simulink model "uavL1G"  (R2018b)
settings: Solver=VariableStepAuto  StartTime=0.0  StopTime=100  RelTol=1e-3
settings Model: Creator=win7-s  LastModifiedBy=JIA X S

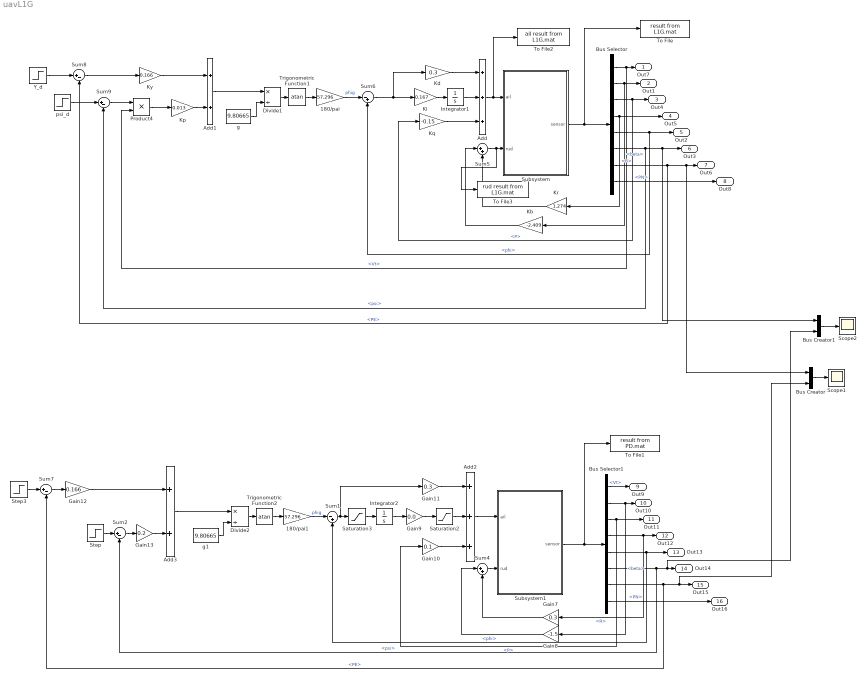
== system uavL1G ==
  180/pai : Gain  Gain=57.296
  180/pai1 : Gain  Gain=57.296
  Add : Sum  Inputs=+++
  Add1 : Sum
  Add2 : Sum  Inputs=+++
  Add3 : Sum
  Bus Creator : BusCreator  Inputs=2
  Bus Creator1 : BusCreator  Inputs=2
  Bus Selector : BusSelector  OutputSignals=Vt,beta,P,R,phi,psi,PE,PN
  Bus Selector1 : BusSelector  OutputSignals=Vt,beta,P,R,phi,psi,PE,PN
  Divide1 : Product  Inputs=*/
  Divide2 : Product  Inputs=*/
  Gain10 : Gain  Gain=0.1
  Gain11 : Gain  Gain=0.3
  Gain12 : Gain  Gain=0.166
  Gain13 : Gain  Gain=0.2
  Gain7 : Gain  Gain=0.3
  Gain8 : Gain  Gain=-1.5
  Gain9 : Gain  Gain=0.0
  Integrator1 : Integrator
  Integrator2 : Integrator
  Kb : Gain  Gain=-2.409
  Kd : Gain  Gain=0.3
  Ki : Gain  Gain=0.167
  Kp : Gain  Gain=0.013
  Kq : Gain  Gain=-0.15
  Kr : Gain  Gain=1.274
  Ky : Gain  Gain=0.166
  Product4 : Product
  Saturation2 : Saturate
  Saturation3 : Saturate
  Scope1 : Scope
  Scope2 : Scope
  Step : Step  Time=0  After=0  SampleTime=0
  Step3 : Step  Time=0  Before=5  After=5  SampleTime=0
  Subsystem : Subsystem
  Subsystem1 : Subsystem
  Sum1 : Sum  Inputs=|-+
  Sum{2,7..9} (4 alike) : Sum  Inputs=|+-
  Sum4 : Sum  Inputs=|++
  Sum5 : Sum  Inputs=|++
  Sum6 : Sum  Inputs=|-+
  To File : ToFile  Filename=result from L1G.mat  SaveFormat=Timeseries
  To File1 : ToFile  Filename=result from PD.mat  SaveFormat=Timeseries
  To File2 : ToFile  Filename=ail result from L1G.mat  SaveFormat=Timeseries
  To File3 : ToFile  Filename=rud result from L1G.mat  SaveFormat=Timeseries
  Trigonometric Function1 : Trigonometry  Operator=atan
  Trigonometric Function2 : Trigonometry  Operator=atan
  Y_d : Step  Time=0  Before=5  After=5  SampleTime=0
  g : Constant  Value=9.80665
  g1 : Constant  Value=9.80665
  psi_d : Step  Time=0  After=0  SampleTime=0
  Out7 : Outport
  Out1 : Outport  Port=2
  Out4 : Outport  Port=3
  Out5 : Outport  Port=4
  Out2 : Outport  Port=5
  Out3 : Outport  Port=6
  Out6 : Outport  Port=7
  Out8 : Outport  Port=8
  Out9 : Outport  Port=9
  Out10 : Outport  Port=10
  Out11 : Outport  Port=11
  Out12 : Outport  Port=12
  Out13 : Outport  Port=13
  Out14 : Outport  Port=14
  Out15 : Outport  Port=15
  Out16 : Outport  Port=16
  wires:
  Bus Selector/7 -> Bus Creator/1, Out6/1, Sum8/2  "<PE>"
  Bus Selector/3 -> Kq/1, Out4/1  "<P>"
  Bus Selector/6 -> Bus Creator1/1, Out3/1, Sum9/2  "<psi>"
  Bus Selector/2 -> Kb/1, Out1/1  "<beta>"
  Bus Selector/5 -> Sum6/2, Out2/1  "<phi>"
  Bus Selector/4 -> Out5/1, Kr/1  "<R>"
  Subsystem/1(sensor) -> To File/1, Bus Selector/1
  g/1 -> Divide1/2
  Divide1/1 -> Trigonometric Function1/1
  Ki/1 -> Integrator1/1
  Bus Selector/1 -> Product4/2, Out7/1  "<Vt>"
  Bus Selector/8 -> Out8/1  "<PN>"
  Integrator1/1 -> Add/2
  Kd/1 -> Add/1
  Kq/1 -> Add/3
  Kb/1 -> Sum5/1
  Kr/1 -> Sum5/2
  Sum6/1 -> Kd/1, Ki/1
  Trigonometric Function1/1 -> 180/pai/1
  Add/1 -> To File2/1, Subsystem/1(ail)
  Sum5/1 -> To File3/1, Subsystem/2(rud)
  Y_d/1 -> Sum8/1
  Ky/1 -> Add1/1
  Product4/1 -> Kp/1
  Sum8/1 -> Ky/1
  Sum9/1 -> Product4/1
  180/pai/1 -> Sum6/1  "phig"
  Kp/1 -> Add1/2
  Add1/1 -> Divide1/1
  psi_d/1 -> Sum9/1
  Bus Selector1/1 -> Out9/1  "<Vt>"
  Bus Selector1/8 -> Out16/1  "<PN>"
  Subsystem1/1(sensor) -> To File1/1, Bus Selector1/1
  Gain13/1 -> Add3/2
  Gain11/1 -> Add2/1
  Gain7/1 -> Sum4/2
  Bus Selector1/3 -> Out11/1, Gain10/1  "<P>"
  Bus Selector1/4 -> Gain7/1, Out12/1  "<R>"
  Gain9/1 -> Saturation2/1
  Sum2/1 -> Gain13/1
  Bus Selector1/6 -> Sum2/2, Bus Creator1/2, Out14/1  "<psi>"
  Bus Selector1/2 -> Gain8/1, Out10/1  "<beta>"
  Gain8/1 -> Sum4/1
  Bus Selector1/5 -> Sum1/2, Out13/1  "<phi>"
  Integrator2/1 -> Gain9/1
  Sum7/1 -> Gain12/1
  Saturation2/1 -> Add2/2
  Saturation3/1 -> Integrator2/1
  Step/1 -> Sum2/1
  Sum4/1 -> Subsystem1/2(rud)
  Gain10/1 -> Add2/3
  Bus Selector1/7 -> Sum7/2, Bus Creator/2, Out15/1  "<PE>"
  Step3/1 -> Sum7/1
  Gain12/1 -> Add3/1
  Sum1/1 -> Gain11/1, Saturation3/1
  Add2/1 -> Subsystem1/1(ail)
  Bus Creator/1 -> Scope1/1
  Bus Creator1/1 -> Scope2/1
  Add3/1 -> Divide2/1
  Trigonometric Function2/1 -> 180/pai1/1
  Divide2/1 -> Trigonometric Function2/1
  g1/1 -> Divide2/2
  180/pai1/1 -> Sum1/1  "phig"

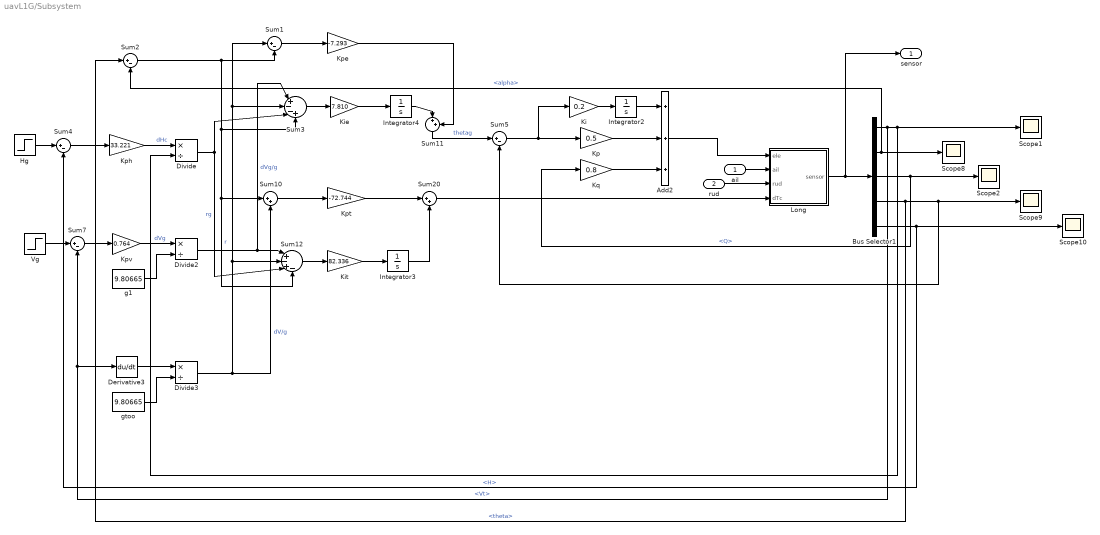
== system uavL1G/Subsystem ==
  ail : Inport
  rud : Inport  Port=2
  Add2 : Sum  Inputs=+++
  Bus Selector1 : BusSelector  OutputSignals=Vt,alpha,Q,theta,H
  Derivative3 : Derivative
  Divide : Product  Inputs=*/
  Divide2 : Product  Inputs=*/
  Divide3 : Product  Inputs=*/
  Hg : Step  Time=0  Before=100  After=100  SampleTime=0
  Integrator2 : Integrator
  Integrator3 : Integrator
  Integrator4 : Integrator
  Ki : Gain  Gain=0.2
  Kie : Gain  Gain=7.810
  Kit : Gain  Gain=82.336
  Kp : Gain  Gain=0.5
  Kpe : Gain  Gain=-7.293
  Kph : Gain  Gain=33.221
  Kpt : Gain  Gain=-72.744
  Kpv : Gain  Gain=0.764
  Kq : Gain  Gain=0.8
  Long : Subsystem
  Scope{1..2,8..10} (5 alike) : Scope
  Sum{1..2,4..5,7} (5 alike) : Sum  Inputs=|+-
  Sum10 : Sum  Inputs=|++
  Sum11 : Sum  Inputs=|++
  Sum12 : Sum  Inputs=|+-+-
  Sum20 : Sum  Inputs=|++
  Sum3 : Sum  Inputs=|+--+
  Vg : Step  Time=0  Before=20  After=20  SampleTime=0
  g1 : Constant  Value=9.80665
  gtoo : Constant  Value=9.80665
  sensor : Outport  VectorParamsAs1DForOutWhenUnconnected=on
  wires:
  Bus Selector1/3 -> Kq/1, Scope2/1  "<Q>"
  Sum10/1 -> Kpt/1
  Kq/1 -> Add2/3
  Divide3/1 -> Sum10/2, Sum12/2, Sum3/2, Sum1/1  "dV/g"
  Sum7/1 -> Kpv/1
  Sum4/1 -> Kph/1
  Integrator3/1 -> Sum20/2
  Bus Selector1/5 -> Sum4/2, Scope10/1  "<H>"
  Hg/1 -> Sum4/1
  Bus Selector1/1 -> Divide/2, Scope1/1, Sum7/2, Derivative3/1  "<Vt>"
  Kph/1 -> Divide/1  "dHc"
  gtoo/1 -> Divide3/2
  Sum1/1 -> Kpe/1
  Divide/1 -> Sum12/3, Sum3/3  "rg"
  Vg/1 -> Sum7/1
  Kpv/1 -> Divide2/1  "dVg"
  Integrator2/1 -> Add2/1
  Bus Selector1/4 -> Sum2/1, Sum5/2, Scope9/1  "<theta>"
  Divide2/1 -> Sum12/1, Sum3/1  "dVg/g"
  Ki/1 -> Integrator2/1
  Sum12/1 -> Kit/1
  Integrator4/1 -> Sum11/1
  Sum3/1 -> Kie/1
  Sum20/1 -> Long/4(dTc)
  Sum11/1 -> Sum5/1  "thetag"
  Derivative3/1 -> Divide3/1
  Kp/1 -> Add2/2
  Kit/1 -> Integrator3/1
  Long/1(sensor) -> sensor/1, Bus Selector1/1
  rud/1 -> Long/3(rud)
  Sum2/1 -> Sum12/4, Sum10/1, Sum3/4, Sum1/2  "r"
  ail/1 -> Long/2(ail)
  Kie/1 -> Integrator4/1
  Sum5/1 -> Ki/1, Kp/1
  Add2/1 -> Long/1(ele)
  Kpt/1 -> Sum20/1
  Bus Selector1/2 -> Scope8/1, Sum2/2  "<alpha>"
  Kpe/1 -> Sum11/2
  g1/1 -> Divide2/2

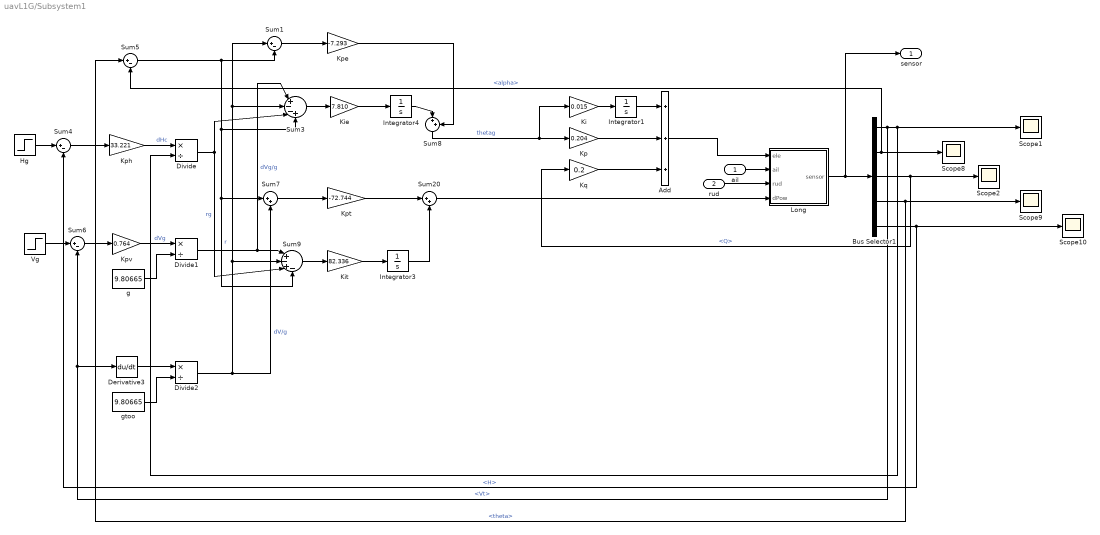
== system uavL1G/Subsystem1 ==
  ail : Inport
  rud : Inport  Port=2
  Add : Sum  Inputs=+++
  Bus Selector1 : BusSelector  OutputSignals=Vt,alpha,Q,theta,H
  Derivative3 : Derivative
  Divide : Product  Inputs=*/
  Divide1 : Product  Inputs=*/
  Divide2 : Product  Inputs=*/
  Hg : Step  Time=0  Before=100  After=100  SampleTime=0
  Integrator1 : Integrator
  Integrator3 : Integrator
  Integrator4 : Integrator
  Ki : Gain  Gain=0.015
  Kie : Gain  Gain=7.810
  Kit : Gain  Gain=82.336
  Kp : Gain  Gain=0.204
  Kpe : Gain  Gain=-7.293
  Kph : Gain  Gain=33.221
  Kpt : Gain  Gain=-72.744
  Kpv : Gain  Gain=0.764
  Kq : Gain  Gain=0.2
  Long : Subsystem
  Scope{1..2,8..10} (5 alike) : Scope
  Sum{1,4..6} (4 alike) : Sum  Inputs=|+-
  Sum20 : Sum  Inputs=|++
  Sum3 : Sum  Inputs=|+--+
  Sum7 : Sum  Inputs=|++
  Sum8 : Sum  Inputs=|++
  Sum9 : Sum  Inputs=|+-+-
  Vg : Step  Time=0  Before=20  After=20  SampleTime=0
  g : Constant  Value=9.80665
  gtoo : Constant  Value=9.80665
  sensor : Outport  VectorParamsAs1DForOutWhenUnconnected=on
  wires:
  Sum6/1 -> Kpv/1
  gtoo/1 -> Divide2/2
  Kie/1 -> Integrator4/1
  Integrator3/1 -> Sum20/2
  Sum8/1 -> Ki/1, Kp/1  "thetag"
  Ki/1 -> Integrator1/1
  Sum1/1 -> Kpe/1
  Sum9/1 -> Kit/1
  Kit/1 -> Integrator3/1
  Vg/1 -> Sum6/1
  Divide2/1 -> Sum7/2, Sum9/2, Sum3/2, Sum1/1  "dV/g"
  Kpv/1 -> Divide1/1  "dVg"
  Kpe/1 -> Sum8/2
  Hg/1 -> Sum4/1
  Divide/1 -> Sum9/3, Sum3/3  "rg"
  Long/1(sensor) -> sensor/1, Bus Selector1/1
  ail/1 -> Long/2(ail)
  Integrator4/1 -> Sum8/1
  Sum5/1 -> Sum9/4, Sum7/1, Sum3/4, Sum1/2  "r"
  Derivative3/1 -> Divide2/1
  rud/1 -> Long/3(rud)
  Divide1/1 -> Sum9/1, Sum3/1  "dVg/g"
  Bus Selector1/4 -> Sum5/1, Scope9/1  "<theta>"
  Sum3/1 -> Kie/1
  g/1 -> Divide1/2
  Sum7/1 -> Kpt/1
  Bus Selector1/1 -> Divide/2, Scope1/1, Sum6/2, Derivative3/1  "<Vt>"
  Kpt/1 -> Sum20/1
  Kph/1 -> Divide/1  "dHc"
  Bus Selector1/5 -> Sum4/2, Scope10/1  "<H>"
  Sum4/1 -> Kph/1
  Bus Selector1/3 -> Kq/1, Scope2/1  "<Q>"
  Sum20/1 -> Long/4(dPow)
  Bus Selector1/2 -> Scope8/1, Sum5/2  "<alpha>"
  Kp/1 -> Add/2
  Add/1 -> Long/1(ele)
  Kq/1 -> Add/3
  Integrator1/1 -> Add/1

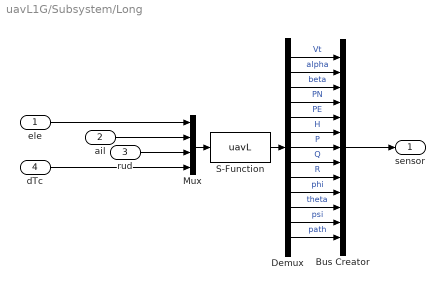
== system uavL1G/Subsystem/Long ==
  ele : Inport
  ail : Inport  Port=2
  rud : Inport  Port=3
  dTc : Inport  Port=4
  Bus Creator : BusCreator  Inputs=13
  Demux : Demux  Outputs=13
  Mux : Mux
  S-Function : S-Function  FunctionName=uavL  SFunctionDeploymentMode=off  EnableBusSupport=off
  sensor : Outport  VectorParamsAs1DForOutWhenUnconnected=on
  wires:
  Bus Creator/1 -> sensor/1
  ele/1 -> Mux/1
  rud/1 -> Mux/3
  Demux/12 -> Bus Creator/12  "psi"
  Mux/1 -> S-Function/1
  ail/1 -> Mux/2
  Demux/10 -> Bus Creator/10  "phi"
  Demux/13 -> Bus Creator/13  "path"
  Demux/5 -> Bus Creator/5  "PE"
  Demux/9 -> Bus Creator/9  "R"
  Demux/8 -> Bus Creator/8  "Q"
  Demux/7 -> Bus Creator/7  "P"
  Demux/6 -> Bus Creator/6  "H"
  Demux/2 -> Bus Creator/2  "alpha"
  Demux/3 -> Bus Creator/3  "beta"
  Demux/11 -> Bus Creator/11  "theta"
  Demux/4 -> Bus Creator/4  "PN"
  Demux/1 -> Bus Creator/1  "Vt"
  dTc/1 -> Mux/4
  S-Function/1 -> Demux/1

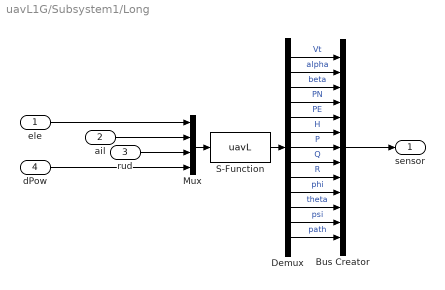
== system uavL1G/Subsystem1/Long ==
  ele : Inport
  ail : Inport  Port=2
  rud : Inport  Port=3
  dPow : Inport  Port=4
  Bus Creator : BusCreator  Inputs=13
  Demux : Demux  Outputs=13
  Mux : Mux
  S-Function : S-Function  FunctionName=uavL  SFunctionDeploymentMode=off  EnableBusSupport=off
  sensor : Outport  VectorParamsAs1DForOutWhenUnconnected=on
  wires:
  Bus Creator/1 -> sensor/1
  ele/1 -> Mux/1
  rud/1 -> Mux/3
  Demux/12 -> Bus Creator/12  "psi"
  Mux/1 -> S-Function/1
  ail/1 -> Mux/2
  Demux/10 -> Bus Creator/10  "phi"
  Demux/13 -> Bus Creator/13  "path"
  Demux/5 -> Bus Creator/5  "PE"
  Demux/9 -> Bus Creator/9  "R"
  Demux/8 -> Bus Creator/8  "Q"
  Demux/7 -> Bus Creator/7  "P"
  Demux/6 -> Bus Creator/6  "H"
  Demux/2 -> Bus Creator/2  "alpha"
  Demux/3 -> Bus Creator/3  "beta"
  Demux/11 -> Bus Creator/11  "theta"
  Demux/4 -> Bus Creator/4  "PN"
  Demux/1 -> Bus Creator/1  "Vt"
  dPow/1 -> Mux/4
  S-Function/1 -> Demux/1
